simulink model "Planta_2"  (Simulink 7.9)
settings: Solver=ode45  StartTime=0.0  StopTime=15  RelTol=1e-3
settings Model: Creator=Carlos  LastModifiedBy=Carlos

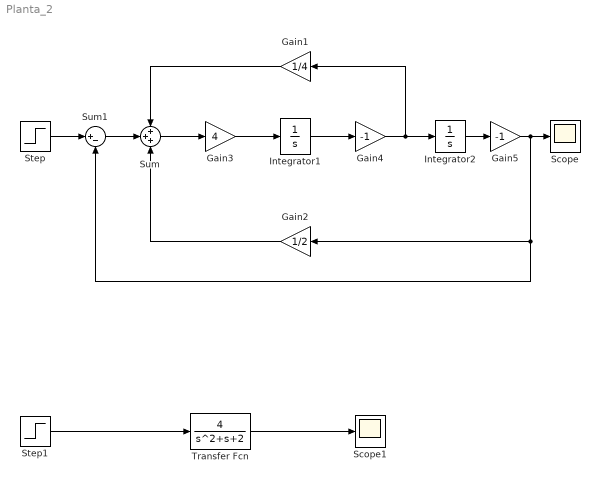
== system Planta_2 ==
  Gain1 : Gain  Gain=1/4
  Gain2 : Gain  Gain=1/2
  Gain3 : Gain  Gain=4
  Gain4 : Gain  Gain=-1
  Gain5 : Gain  Gain=-1
  Integrator1 : Integrator  LimitOutput=on  UpperSaturationLimit=10.5  LowerSaturationLimit=-10.5
  Integrator2 : Integrator  LimitOutput=on  UpperSaturationLimit=10.5  LowerSaturationLimit=-10.5
  Scope : Scope
  Scope1 : Scope
  Step : Step  Time=0.01  SampleTime=0
  Step1 : Step  Time=0.01  SampleTime=0
  Sum : Sum  Inputs=+++
  Sum1 : Sum  Inputs=|+-
  Transfer Fcn : TransferFcn  Numerator=[4]  Denominator=[1 1 2]
  wires:
  Sum/1 -> Gain3/1
  Gain1/1 -> Sum/1
  Gain2/1 -> Sum/3
  Gain3/1 -> Integrator1/1
  Integrator1/1 -> Gain4/1
  Gain4/1 -> Integrator2/1, Gain1/1
  Integrator2/1 -> Gain5/1
  Gain5/1 -> Scope/1, Gain2/1, Sum1/2
  Step1/1 -> Transfer Fcn/1
  Transfer Fcn/1 -> Scope1/1
  Sum1/1 -> Sum/2
  Step/1 -> Sum1/1
